simulink model "vehstlin_mdl_callback_mask2_inout"  (R2021b)
settings: Solver=ode45  StartTime=0.0  StopTime=14  MaxStep=1e-3  MinStep=1e-4  RelTol=1e-3  AbsTol=1e-6
StartFcn:
  | disp('Starting model...');
StopFcn:
  | % Set limits of XY Graph according to simulation
  | block = [bdroot, '/Path'];
  | rto = get_param(block,'RuntimeObject');
  | xmax = rto.InputPort(1).Data;
  | ymax = rto.InputPort(2).Data;
  | set_param(block, 'xmax', num2str(xmax));
  | set_param(block, 'ymax', num2str(ymax));
  | 
  | disp('Stopping model...');
values from neighbouring files (symbols this model uses):
  A = [a11, 0, a13, 0 ... (first row only)    [vehstlin_sseval.m]
  B = [b11 ... (first row only)    [vehstlin_sseval.m]
  C = [0, 0, 1, 0]    [vehstlin_sseval.m]
  c_f = 16.32    [vehstlin_param.m]
  c_r = 18.45    [vehstlin_param.m]
  D = 0    [vehstlin_sseval.m]
  J = 2230    [vehstlin_param.m]
  l_f = 1.268    [vehstlin_param.m]
  l_r = 1.62    [vehstlin_param.m]
  m = 1564    [vehstlin_param.m]
  v = 20    [vehstlin_param.m]
undefined symbols (not defined in the file or in its folder): vehstlin_param
settings Model: Creator=hfe2bp  LastModifiedBy=Lindenmaier László
settings SolverCC: AutoScaleAbsTol=off  InitialStep=1e-3  AlgebraicLoopSolver=TrustRegion
settings DataIOCC: ExternalInput=[t_in, u_in]  LoadExternalInput=on  SaveFormat=Array  SignalLogging=off  DSMLogging=off  ReturnWorkspaceOutputs=off  TimeSaveName=t_out  OutputSaveName=y_out
settings DebuggingCC: SFMachineParentedDataDiag=warning  ArithmeticOperatorsInVariantConditions=warning
settings SFSimCC: SimUseLocalCustomCode=off  CustomCodeUndefinedFunction=UseInterfaceOnly
settings RTWCC: RTWUseLocalCustomCode=off
settings CodeAppCC: StateflowObjectComments=on

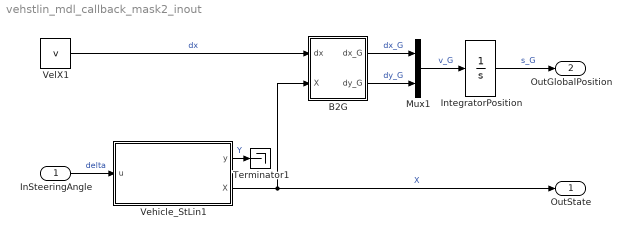
== system vehstlin_mdl_callback_mask2_inout ==
  InSteeringAngle : Inport
  B2G : Subsystem
  IntegratorPosition : Integrator
  Mux1 : Mux  Inputs=2
  Terminator1 : Terminator
  Vehicle_StLin1 : Subsystem  InitFcn=vehstlin_param;  mask(LTI){m=m, v=v, c_f=c_f, c_r=c_r, l_f=l_f, l_r=l_r, J=J}
      mask prompts: m "Gross vehicle mass"; v "Longitudinal velocity"; c_f "Cornering stiffness front"; c_r "Cornering stiffness rear"; l_f "Center of gravity distance front"; l_r "Center of gravity distance rear"; J "Moment of intertia about vertical axis"
      mask help: State space representation of a linear time-invariant system.
      mask init:
      | [A, B, C, D] = vehstlin_sseval(m, J, v, c_f, c_r, l_f, l_r);
      mask Display:
      | image('vehstlin_icon.png');
      | port_label('input', 1, 'delta_f');
      | port_label('output', 1, 'dpsi');
      | port_label('output', 2, 'X');
  VelX1 : Constant  Value=v
  OutState : Outport  VectorParamsAs1DForOutWhenUnconnected=off
  OutGlobalPosition : Outport  Port=2  VectorParamsAs1DForOutWhenUnconnected=off
  wires:
  InSteeringAngle/1 -> Vehicle_StLin1/1(u)  "delta"
  Vehicle_StLin1/1(y) -> Terminator1/1  "Y"
  VelX1/1 -> B2G/1(dx)  "dx"
  B2G/1(dx_G) -> Mux1/1  "dx_G"
  B2G/2(dy_G) -> Mux1/2  "dy_G"
  Mux1/1 -> IntegratorPosition/1  "v_G"
  IntegratorPosition/1 -> OutGlobalPosition/1  "s_G"
  Vehicle_StLin1/2(X) -> OutState/1, B2G/2(X)  "X"

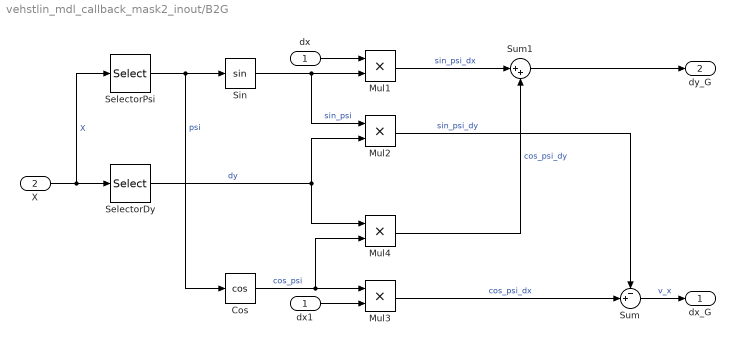
== system vehstlin_mdl_callback_mask2_inout/B2G ==
  dx : Inport
  X : Inport  Port=2
  Cos : Trigonometry  Operator=cos
  Mul{1..4} (4 alike) : Product  Inputs=**
  SelectorDy : Selector  InputPortWidth=4  IndexOptions=Index vector (dialog)  Indices=[1]  OutputSizes=1
  SelectorPsi : Selector  InputPortWidth=4  IndexOptions=Index vector (dialog)  Indices=[4]  OutputSizes=1
  Sin : Trigonometry
  Sum : Sum  Inputs=-+|
  Sum1 : Sum  Inputs=|++
  dx1 : InportShadow
  dx_G : Outport  VectorParamsAs1DForOutWhenUnconnected=off
  dy_G : Outport  Port=2  VectorParamsAs1DForOutWhenUnconnected=off
  wires:
  Cos/1 -> Mul4/2, Mul3/1  "cos_psi"
  Sin/1 -> Mul2/1, Mul1/2  "sin_psi"
  SelectorPsi/1 -> Cos/1, Sin/1  "psi"
  X/1 -> SelectorPsi/1, SelectorDy/1  "X"
  SelectorDy/1 -> Mul4/1, Mul2/2  "dy"
  dx/1 -> Mul1/1
  dx1/1 -> Mul3/2
  Mul1/1 -> Sum1/1  "sin_psi_dx"
  Mul2/1 -> Sum/1  "sin_psi_dy"
  Mul4/1 -> Sum1/2  "cos_psi_dy"
  Mul3/1 -> Sum/2  "cos_psi_dx"
  Sum/1 -> dx_G/1  "v_x"
  Sum1/1 -> dy_G/1

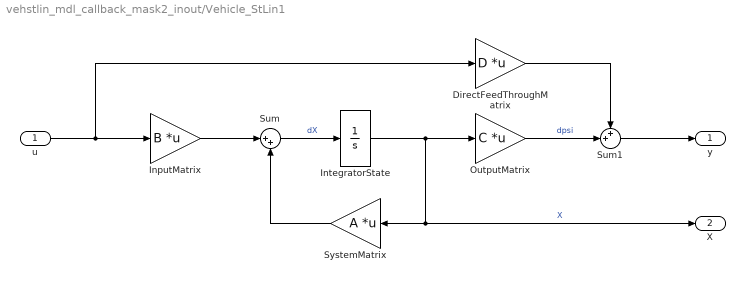
== system vehstlin_mdl_callback_mask2_inout/Vehicle_StLin1 ==
  u : Inport
  DirectFeedThroughMatrix : Gain  Gain=D  Multiplication=Matrix(K*u)
  InputMatrix : Gain  Gain=B  Multiplication=Matrix(K*u)
  IntegratorState : Integrator
  OutputMatrix : Gain  Gain=C  Multiplication=Matrix(K*u)
  Sum : Sum  Inputs=|++
  Sum1 : Sum  Inputs=++|
  SystemMatrix : Gain  Gain=A  Multiplication=Matrix(K*u)
  y : Outport  VectorParamsAs1DForOutWhenUnconnected=off
  X : Outport  Port=2  VectorParamsAs1DForOutWhenUnconnected=off
  wires:
  DirectFeedThroughMatrix/1 -> Sum1/1
  Sum1/1 -> y/1
  OutputMatrix/1 -> Sum1/2  "dpsi"
  u/1 -> DirectFeedThroughMatrix/1, InputMatrix/1
  InputMatrix/1 -> Sum/1
  SystemMatrix/1 -> Sum/2
  IntegratorState/1 -> OutputMatrix/1, SystemMatrix/1, X/1  "X"
  Sum/1 -> IntegratorState/1  "dX"
